simulink model "test_10gbe_pkt_src_sim"  (Simulink 6.2)
settings: Solver=ode45  StartTime=0.0  StopTime=20000  RelTol=1e-3
libraries: xbsIndex_r3 x30, xps_library x6, casper_library x2
settings Model: LastModifiedBy=dsp
settings DebuggingCC: SolverPrmCheckMsg=warning

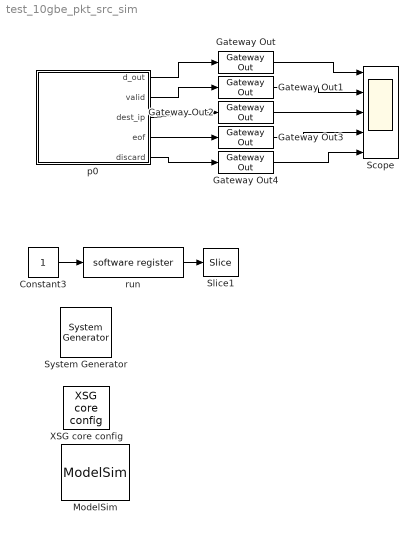
== system test_10gbe_pkt_src_sim ==
  " System Generator" : xbsIndex_r3/ System Generator  Tag=genX  xilinxfamily=Virtex2P  part=xc2vp70  speed=-7  package=ff1704  synthesis_tool=XST  directory=./b_2x_8a_r308d/sysgen  testbench=off  simulink_period=1  sysclk_period=4.878  incr_netlist=off  trim_vbits=Everywhere in SubSystem  dbl_ovrd=According to Block Masks  core_generation=According to Block Masks  run_coregen=off  deprecated_control=off  eval_field=0
      settings: AttributesFormatString=System\nGenerator
  Constant3 : Constant
  Gateway Out{,1..4} (5 alike) : xbsIndex_r3/Gateway Out  output_type=Double  nbits=8  bin_pt=6  arith_type=Boolean  quantization=Truncate  overflow=Wrap  hdl_port=on  timing_constraint=None  locs_specified=off  LOCs={}  needs_fixed_name=off  show_param=off
      settings: xl_area=[0, 0, 0, 0, 0, 0, 0]
  ModelSim : xbsIndex_r3/ModelSim  dir=./modelsim  waveform=on  leave_open=on  skip_compile=off  custom_scripts=off  startup_timeout=40
  Scope : Scope  NumInputPorts=5
      settings: YMin=1500~0~1.67772e+008~0~-1  YMax=3000~1~1.67772e+008~1~1
  Slice1 : xbsIndex_r3/Slice  mode=Lower Bit Location + Width  nbits=1  bit1=1  base1=MSB of Input  bit0=0  base0=LSB of Input  boolean_output=off  explicit_period=off  period=1  dbl_ovrd=off
  XSG core config : xps_library/XSG core config  Tag=xps:xsg  hw_sys=BEE2_usr  ibob_linux=off  clk_src=sys_clk2x  gpio_clk_io_group=iBOB:sma  gpio_clk_bit_index=0  clk_rate=205  sample_period=1  synthesis_tool=XST  mpc_type=powerpc405
  p0 : Subsystem
  run : xps_library/software register  Tag=xps:sw_reg  io_dir=From Processor  arith_type=Unsigned  bitwidth=32  bin_pt=0  sample_period=1  gw_name=test_10gbe_pkt_src_sim_run_user_data_out
  wires:
  Gateway Out/1 -> Scope/1
  Gateway Out1/1 -> Scope/2
  Gateway Out2/1 -> Scope/3
  Gateway Out3/1 -> Scope/4
  Gateway Out4/1 -> Scope/5
  p0/1(d_out) -> Gateway Out/1
  p0/2(valid) -> Gateway Out1/1
  p0/3(dest_ip) -> Gateway Out2/1
  p0/4(eof) -> Gateway Out3/1
  p0/5(discard) -> Gateway Out4/1
  Constant3/1 -> run/1
  run/1 -> Slice1/1

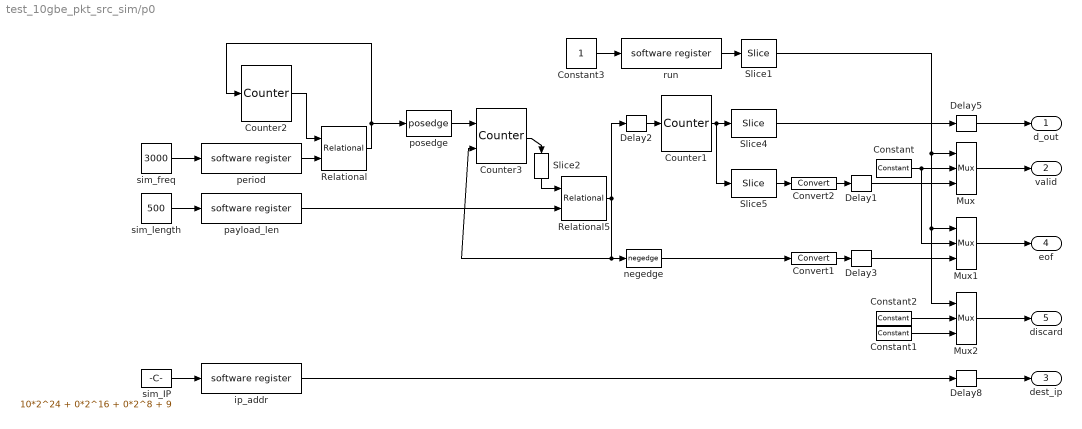
== system test_10gbe_pkt_src_sim/p0 ==
  Constant : xbsIndex_r3/Constant  const=0  equ=P=C  arith_type=Boolean  n_bits=1  bin_pt=0  opselect=C  inp2=PCIN>>17  opr=+  inp1=P  carry=CIN  iostate=0  explicit_period=on  period=1  dbl_ovrd=off
  Constant1 : xbsIndex_r3/Constant  const=0  equ=P=C  arith_type=Boolean  n_bits=1  bin_pt=0  opselect=C  inp2=PCIN>>17  opr=+  inp1=P  carry=CIN  iostate=0  explicit_period=on  period=1  dbl_ovrd=off
  Constant2 : xbsIndex_r3/Constant  const=1  equ=P=C  arith_type=Boolean  n_bits=1  bin_pt=0  opselect=C  inp2=PCIN>>17  opr=+  inp1=P  carry=CIN  iostate=0  explicit_period=on  period=1  dbl_ovrd=off
  Constant3 : Constant
  Convert1 : xbsIndex_r3/Convert  arith_type=Boolean  n_bits=8  bin_pt=6  quantization=Truncate  overflow=Wrap  latency=0  explicit_period=on  period=1  dbl_ovrd=off  show_param=off  inserted_by_tool=off  pipeline=off
      settings: xl_area=[0, 0, 0, 0, 0, 0, 0]
  Convert2 : xbsIndex_r3/Convert  arith_type=Boolean  n_bits=8  bin_pt=6  quantization=Truncate  overflow=Wrap  latency=0  explicit_period=on  period=1  dbl_ovrd=off  show_param=off  inserted_by_tool=off  pipeline=off
      settings: xl_area=[0, 0, 0, 0, 0, 0, 0]
  Counter1 : xbsIndex_r3/Counter  cnt_type=Free Running  n_bits=65  bin_pt=0  arith_type=Unsigned  start_count=0  cnt_to=Inf  cnt_by_val=1  operation=Up  explicit_period=off  period=1  load_pin=off  rst=off  en=on  dbl_ovrd=off  show_param=off  use_rpm=off  gen_core=off
      settings: xl_area=[0, 0, 0, 0, 0, 0, 0]
  Counter2 : xbsIndex_r3/Counter  cnt_type=Free Running  n_bits=32  bin_pt=0  arith_type=Unsigned  start_count=0  cnt_to=Inf  cnt_by_val=1  operation=Up  explicit_period=on  period=1  load_pin=off  rst=on  en=off  dbl_ovrd=off  show_param=off  use_rpm=on  gen_core=off
      settings: xl_area=[0, 0, 0, 0, 0, 0, 0]
  Counter3 : xbsIndex_r3/Counter  cnt_type=Free Running  n_bits=33  bin_pt=0  arith_type=Unsigned  start_count=0  cnt_to=1023  cnt_by_val=1  operation=Up  explicit_period=on  period=1  load_pin=off  rst=on  en=on  dbl_ovrd=off  show_param=off  use_rpm=on  gen_core=off
      settings: xl_area=[0, 0, 0, 0, 0, 0, 0]
  Delay{1..3,5,8} (5 alike) : xbsIndex_r3/Delay  latency=1  reg_retiming=on  explicit_period=off  period=1  en=off  accept_only_valid=off  init_zero=on  dbl_ovrd=off  show_param=off
      settings: xl_area=[0, 0, 0, 0, 0, 0, 0]
  Mux : xbsIndex_r3/Mux  inputs=2  precision=Full  arith_type="Signed  (2's comp)"  n_bits=8  bin_pt=2  quantization=Truncate  overflow=Wrap  latency=1  explicit_period=off  period=1  en=off  dbl_ovrd=off  show_param=off  mux_type=off  use_rpm=off  gen_core=off
      settings: xl_area=[0, 0, 0, 0, 0, 0, 0]
  Mux1 : xbsIndex_r3/Mux  inputs=2  precision=Full  arith_type="Signed  (2's comp)"  n_bits=8  bin_pt=2  quantization=Truncate  overflow=Wrap  latency=1  explicit_period=off  period=1  en=off  dbl_ovrd=off  show_param=off  mux_type=off  use_rpm=off  gen_core=off
      settings: xl_area=[0, 0, 0, 0, 0, 0, 0]
  Mux2 : xbsIndex_r3/Mux  inputs=2  precision=Full  arith_type="Signed  (2's comp)"  n_bits=8  bin_pt=2  quantization=Truncate  overflow=Wrap  latency=1  explicit_period=off  period=1  en=off  dbl_ovrd=off  show_param=off  mux_type=off  use_rpm=off  gen_core=off
      settings: xl_area=[0, 0, 0, 0, 0, 0, 0]
  Relational : xbsIndex_r3/Relational  mode=a=b  latency=1  explicit_period=on  period=1  en=off  dbl_ovrd=off  show_param=off
      settings: xl_area=[0, 0, 0, 0, 0, 0, 0]
  Relational5 : xbsIndex_r3/Relational  mode=a<b  latency=0  explicit_period=off  period=1  en=off  dbl_ovrd=off  show_param=off
      settings: xl_area=[0, 0, 0, 0, 0, 0, 0]
  Slice1 : xbsIndex_r3/Slice  mode=Lower Bit Location + Width  nbits=1  bit1=1  base1=MSB of Input  bit0=0  base0=LSB of Input  boolean_output=off  explicit_period=off  period=1  dbl_ovrd=off
  Slice2 : xbsIndex_r3/Slice  Orientation=down  mode=Lower Bit Location + Width  nbits=32  bit1=0  base1=MSB of Input  bit0=1  base0=LSB of Input  boolean_output=off  explicit_period=on  period=1  dbl_ovrd=off
  Slice4 : xbsIndex_r3/Slice  mode=Upper Bit Location + Width  nbits=64  bit1=0  base1=MSB of Input  bit0=0  base0=LSB of Input  boolean_output=off  explicit_period=on  period=1  dbl_ovrd=off
  Slice5 : xbsIndex_r3/Slice  mode=Lower Bit Location + Width  nbits=1  bit1=1  base1=MSB of Input  bit0=0  base0=LSB of Input  boolean_output=off  explicit_period=off  period=1  dbl_ovrd=off
  ip_addr : xps_library/software register  Tag=xps:sw_reg  io_dir=From Processor  arith_type=Unsigned  bitwidth=32  bin_pt=0  sample_period=1  gw_name=test_10gbe_pkt_src_sim_p0_ip_addr_user_data_out
  negedge : casper_library/Misc/negedge  Tag=Rising Edge Detector
  payload_len : xps_library/software register  Tag=xps:sw_reg  io_dir=From Processor  arith_type=Unsigned  bitwidth=32  bin_pt=0  sample_period=1  gw_name=test_10gbe_pkt_src_sim_p0_payload_len_user_data_out
  period : xps_library/software register  Tag=xps:sw_reg  io_dir=From Processor  arith_type=Unsigned  bitwidth=32  bin_pt=0  sample_period=1  gw_name=test_10gbe_pkt_src_sim_p0_period_user_data_out
  posedge : casper_library/Misc/pulse_ext/posedge  Tag=Rising Edge Detector
  run : xps_library/software register  Tag=xps:sw_reg  io_dir=From Processor  arith_type=Unsigned  bitwidth=32  bin_pt=0  sample_period=1  gw_name=test_10gbe_pkt_src_sim_p0_run_user_data_out
  sim_IP : Constant  Value=10*2^24 + 0*2^16 + 0*2^8 + 9
  sim_freq : Constant  Value=3000
  sim_length : Constant  Value=500
  d_out : Outport
  valid : Outport  Port=2
  dest_ip : Outport  Port=3
  eof : Outport  Port=4
  discard : Outport  Port=5
  wires:
  Counter1/1 -> Slice4/1, Slice5/1
  Slice5/1 -> Convert2/1
  Convert2/1 -> Delay1/1
  Delay2/1 -> Counter1/1
  negedge/1 -> Convert1/1
  Slice4/1 -> Delay5/1
  Mux/1 -> valid/1
  Constant/1 -> Mux/2, Mux1/2
  Delay1/1 -> Mux/3
  Mux1/1 -> eof/1
  Constant2/1 -> Mux2/2
  Constant1/1 -> Mux2/3
  Convert1/1 -> Delay3/1
  Delay5/1 -> d_out/1
  Delay8/1 -> dest_ip/1
  Delay3/1 -> Mux1/3
  Counter2/1 -> Relational/1
  Relational/1 -> Counter2/1, posedge/1
  period/1 -> Relational/2
  ip_addr/1 -> Delay8/1
  Relational5/1 -> Counter3/2, negedge/1, Delay2/1
  Counter3/1 -> Slice2/1
  posedge/1 -> Counter3/1
  payload_len/1 -> Relational5/2
  Slice1/1 -> Mux/1, Mux1/1, Mux2/1
  Mux2/1 -> discard/1
  Slice2/1 -> Relational5/1
  sim_IP/1 -> ip_addr/1
  sim_length/1 -> payload_len/1
  sim_freq/1 -> period/1
  run/1 -> Slice1/1
  Constant3/1 -> run/1
